simulink model "exam6_sim"  (R2023a)
settings: Solver=VariableStepAuto  StartTime=0.0  StopTime=10.0  RelTol=1e-9
values from neighbouring files (symbols this model uses):
  K = (A*pi*w)/(2*M)    (= 7.85398163397)    [exam6.m]
  M = 8    [exam5.m]    (also in exam6.m = 10)
libraries: cstblocks x1
settings Model: Creator=laptop  LastModifiedBy=laptop

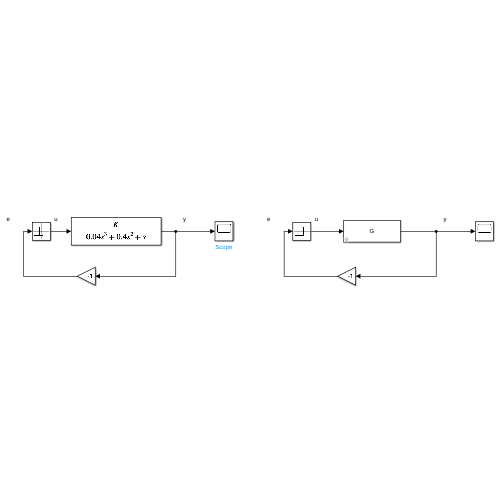
[thumbnail: Simulink's stored preview of the top-level diagram]
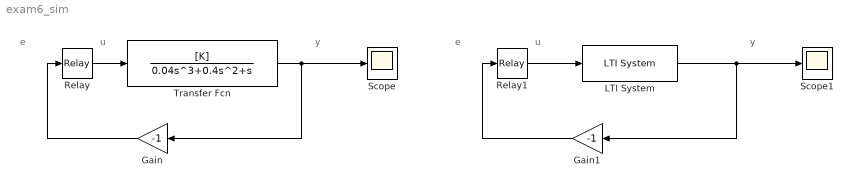
== system exam6_sim ==
  note: e
  note: y
  note: u
  note: y
  note: u
  note: e
  Gain : Gain  Gain=-1
  Gain1 : Gain  Gain=-1
  LTI System : cstblocks/LTI System  sys=G  IC=[]
  Relay : Relay  OnSwitchValue=0  OffSwitchValue=0  OnOutputValue=M  OffOutputValue=-M
  Relay1 : Relay  OnSwitchValue=0  OffSwitchValue=0  OnOutputValue=M  OffOutputValue=-M
  Scope : Scope
  Scope1 : Scope
  Transfer Fcn : TransferFcn  Numerator=[K]  Denominator=[0.04 0.4 1 0]
  wires:
  Relay/1 -> Transfer Fcn/1
  Transfer Fcn/1 -> Gain/1, Scope/1
  Gain/1 -> Relay/1
  Gain1/1 -> Relay1/1
  Relay1/1 -> LTI System/1
  LTI System/1 -> Gain1/1, Scope1/1
